simulink model "Car"  (R2016b)
settings: Solver=FixedStepAuto  StartTime=0.0  StopTime=10.0  RelTol=1e-3
settings Model: Creator=NEATdemo  LastModifiedBy=NEATdemo

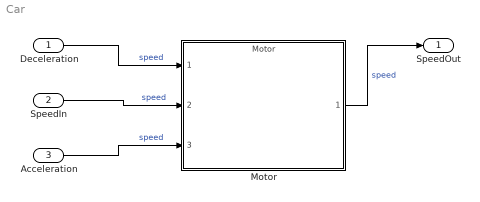
== system Car ==
  Deceleration : Inport
      settings: AttributesFormatString=speed
  SpeedIn : Inport  Port=2
      settings: AttributesFormatString=speed
  Acceleration : Inport  Port=3
      settings: AttributesFormatString=speed
  Motor : ModelReference  ModelNameDialog=Motor  SimulationMode=Normal  ModelReferenceVersion=1.3
  SpeedOut : Outport
      settings: AttributesFormatString=speed
  wires:
  Acceleration/1 -> Motor/3  "speed"
  Deceleration/1 -> Motor/1  "speed"
  Motor/1 -> SpeedOut/1  "speed"
  SpeedIn/1 -> Motor/2  "speed"
